simulink model "simple"  (R2024b)
settings: Solver=VariableStepAuto  StartTime=0.0  StopTime=10.0  RelTol=1e-3
values from neighbouring files (symbols this model uses):
  g = 9.81    [Simple_Pendulum_Motion_Simulation.m]    (also in Simple_Pendulum_Motion_Simulation_code.m)
  L = 1    [Simple_Pendulum_Motion_Simulation.m]    (also in Simple_Pendulum_Motion_Simulation_code.m = i)
settings Model: Creator=Ahmad  LastModifiedBy=Ahmad

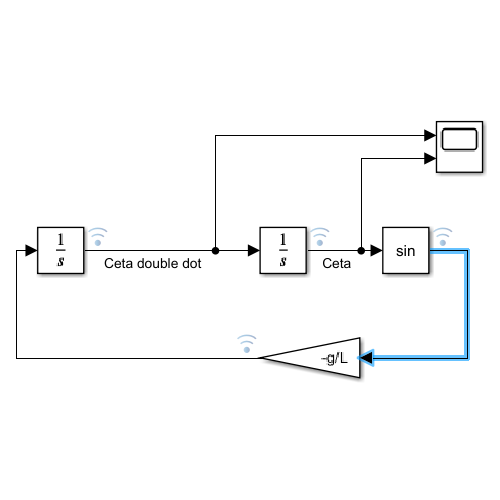
[thumbnail: Simulink's stored preview of the top-level diagram]
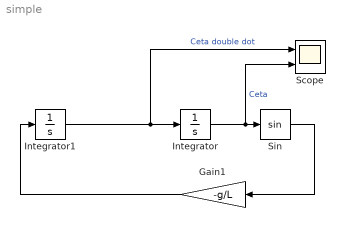
== system simple ==
  Gain1 : Gain  Gain=-g/L
  Integrator : Integrator  InitialCondition=1
  Integrator1 : Integrator
  Scope : Scope  NumInputPorts=2
  Sin : Trigonometry
  wires:
  Sin/1 -> Gain1/1
  Integrator/1 -> Scope/2, Sin/1  "Ceta"
  Integrator1/1 -> Scope/1, Integrator/1  "Ceta double dot"
  Gain1/1 -> Integrator1/1
